simulink model "mobile_gravite"  (R2023a)
settings: Solver=VariableStepAuto  StartTime=0.0  StopTime=10.0  RelTol=1e-3
settings Model: Creator=ave9761  LastModifiedBy=ave9761

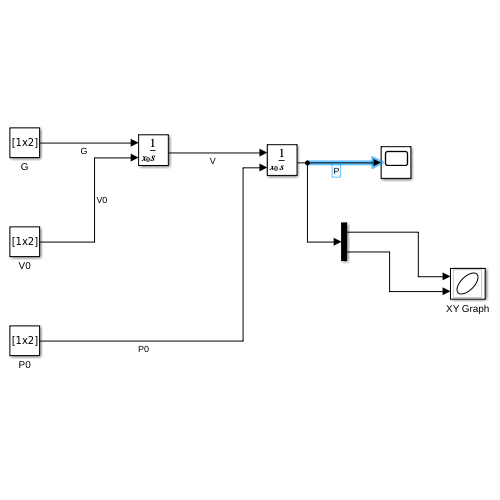
[thumbnail: Simulink's stored preview of the top-level diagram]
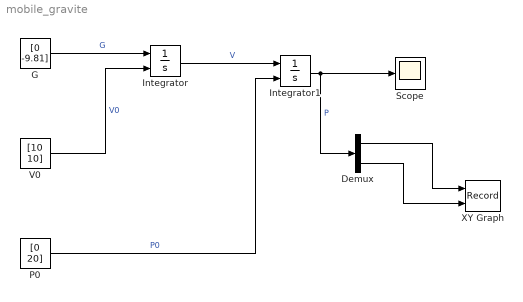
== system mobile_gravite ==
  Demux : Demux  Outputs=2
  G : Constant  Value=[0 -9.81]
  Integrator : Integrator  InitialConditionSource=external
  Integrator1 : Integrator  InitialConditionSource=external
  P0 : Constant  Value=[0 20]
  Scope : Scope
  V0 : Constant  Value=[10 10]
  XY Graph : Record  FileSettingsInternal="{\"entries\":[{\"content\":{\"excelSettings\":{\"content\":{},\"type\":\"Streamout.ExcelSettings\"}},\"type\":\"Streamout.FileSettingStorage\",\"uuid\":\"638bbe18-9bcf-4a60-beb2-4052db86543c\"}],\"packageUris\":[\"http://schema.mathworks.com/mf0/streamout_blocks/R2020a\"],\"version\":\"1.0\"}"  Layout=[1 1]  SignalsInternal="{\"entries\":[{\"content\":{\"signals\":[{\"content\":{\"blockPath\":[\"mobile_gravite/XY Graph\"],\"dimensions\":[1],\"domain\":\"mobile_gravite/XY Graph\",\"lineColor\":\"#a2142f\",\"plots\":[1],\"port\":1,\"sid\":[\"\"],\"signalID\":35,\"signalName\":\"Demux:1\"},\"type\":\"RecordBlkView.Signal\",\"uuid\":\"f3fa203a-ad61-4658-9237-3dc1b1896893\"},{\"content\":{\"blockPath\":[\"mobile_gravite/XY Graph\"],\"dimensions\":[1],\"domain\":\"mobile_gravite/XY Graph\",\"lineColor\":\"#139fff\",\"plots\":[1],\"port\":2,\"sid\":[\"\"],\"signalID\":39,\"signalName\":\"Demux:2\"},\"type\":\"RecordBlkView.Signal\",\"uuid\":\"d24ccf5a-7091-4380-bb34-2bf2e5c7cd2b\"}]},\"type\":\"RecordBlkView.InputSignals\",\"uuid\":\"6104fede-51e7-4f0d-b9f1-cce512a4eebd\"}],\"packageUris\":[\"http://schema.mathworks.com/mf0/streamout_blocks/R2020a\"],\"version\":\"1.0\"}"  VisualizationBindings="{\"xyplotplugin\":{\"info\":[{\"series\":[{\"bindingParametersList\":[{\"parameter\":\"X-Axis\",\"signalID\":35,\"signalName\":\"Demux:1\"},{\"parameter\":\"Y-Axis\",\"signalID\":39,\"signalName\":\"Demux:2\"}],\"seriesID\":48680}],\"subplotID\":1}]}}"  CompatibilityTag=XY
  wires:
  G/1 -> Integrator/1  "G"
  Integrator/1 -> Integrator1/1  "V"
  V0/1 -> Integrator/2  "V0"
  P0/1 -> Integrator1/2  "P0"
  Integrator1/1 -> Demux/1, Scope/1  "P"
  Demux/1 -> XY Graph/1
  Demux/2 -> XY Graph/2
